simulink library "lib"  (R2020a)
settings: Solver=VariableStepAuto  StartTime=0.0  StopTime=10.0  RelTol=1e-3
settings Model: Creator=sreeram  LastModifiedBy=sreeram

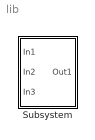
== system lib ==
  Subsystem : Subsystem  mask{A=0, B=0, N=0}

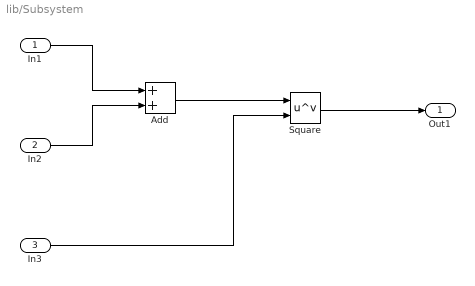
== system lib/Subsystem ==
  In1 : Inport
  In2 : Inport  Port=2
  In3 : Inport  Port=3
  Add : Sum
  Square : Math  Operator=pow  SaturateOnIntegerOverflow=on
  Out1 : Outport
  wires:
  Add/1 -> Square/1
  In1/1 -> Add/1
  Square/1 -> Out1/1
  In2/1 -> Add/2
  In3/1 -> Square/2
